simulink model "sgm_iox_io397_pwm_motor_control"  (R2018a)
settings: Solver=FixedStepDiscrete  StartTime=0.0  StopTime=inf  FixedStep=0.001  RelTol=1e-3  EnableMultiTasking=on
undefined symbols (not defined in the file): IO397
libraries: simulink x2, speedgoatlib_fpga_analog_io x1, speedgoatlib_fpga_pwm x1, speedgoatlib_fpga x1
settings Model: SimulationMode=external  ExtModeArmWhenConnect=off  Creator=deastman  LastModifiedBy=daniel.fonte
settings SolverCC: ConcurrentTasks=on  PositivePriorityOrder=on  AutoInsertRateTranBlk=on
settings DataIOCC: LimitDataPoints=on  SaveFormat=StructureWithTime
settings OptimizationCC: BlockReduction=off  OptimizeBlockIOStorage=off  BufferReuse=off  GlobalBufferReuse=off  ExpressionFolding=off  ExpressionDepthLimit=2147483647  LocalBlockOutputs=off  OptimizeDataStoreBuffers=off  BusAssignmentInplaceUpdate=off
settings DebuggingCC: UnderspecifiedInitializationDetection=Classic  MergeDetectMultiDrivingBlocksExec=none  SolverPrmCheckMsg=warning  FcnCallInpInsideContextMsg=warning  AllowSymbolicDim=off  StateNameClashWarn=warning  SFUnexpectedBacktrackingDiag=warning  SFNoUnconditionalDefaultTransitionDiag=warning  SFExecutionAtInitializationDiag=none
settings HardwareCC: ProdBitPerPointer=32  ProdBitPerSizeT=32  ProdBitPerPtrDiffT=32  ProdLargestAtomicFloat=None  ProdWordSize=32  ProdLongLongMode=on  ProdHWDeviceType=Generic->32-bit x86 compatible
settings ModelReferenceCC: PropagateSignalLabelsOutOfModel=off
settings RTWCC: SystemTargetFile=slrt.tlc  TemplateMakefile=slrt_default_tmf  Description=Simulink Real-Time  RTWVerbose=off  Toolchain=Simulink Real-Time Toolchain  BuildConfiguration=Faster Runs  CodeExecutionProfiling=on  RTWCompilerOptimization=on
settings CodeAppCC: StateflowObjectComments=on
settings SimulinkRealTimeCC: SupportVariableSizeSignals=on  RL32LogTETModifier=off  xPCConcurrentTasks=on
settings ConfigComp: CovMetricSettings=dw  CovSaveCumulativeToWorkspaceVar=on  CovSaveSingleToWorkspaceVar=on  CovExternalEMLEnable=off  CovSFcnEnable=off

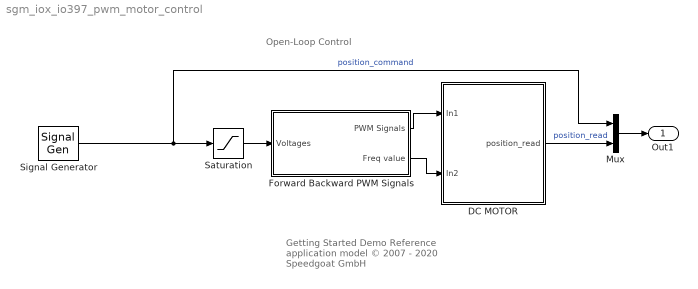
== system sgm_iox_io397_pwm_motor_control ==
  note: Open-Loop Control
  note: Getting Started Demo
      | Reference application model
      | © 2007 - 2020 Speedgoat GmbH
  DC MOTOR : Subsystem
      mask Display: image(imread('hs422.jpg'))
  Forward Backward PWM Signals : Subsystem
      mask init:
      | wave = sin(0:0.4:12);
      | a = length(wave);
      | x1 = linspace(0,8,a);
      | nan1 = NaN(1,2);
      | x2 = x1(end)+[0 1];
      | arrowY = [0 0 0.16 NaN -0.16 0];
      | x3 = x2(end)+[0 2 1.6 NaN 1.6 2];
      | nan2 = NaN(1,2);
      | x4 = x3(end)+[0 1];
      | squareY = [0.5 0 0 0.5 0.5 0 0 0.5 0.5 0 0 0.5 0.5 0 0 0.5 0.5 0 0 0.5 0.5 0];
      | x5 = x4(end)+[0 0 0.4 0.4 0.9 0.9 2.3 2.3 2.6 2.6 3.1 3.1 4.7 4.7 5.4 5.4 5.8 5.8 7.3 7.3 8 8];
      mask Display: plot([x1 x2 x3 x4 x5],[wave nan1 arrowY nan2 squareY])
  Mux : Mux  Inputs=2
  Saturation : Saturate  UpperLimit=5  LowerLimit=-5
  Signal Generator : SignalGenerator  WaveForm=square  Frequency=0.5
  Out1 : Outport
  wires:
  Saturation/1 -> Forward Backward PWM Signals/1(Voltages)
  Forward Backward PWM Signals/1(PWM Signals) -> DC MOTOR/1(In1)
  Mux/1 -> Out1/1
  DC MOTOR/1(position_read) -> Mux/2  "position_read"
  Signal Generator/1 -> Mux/1, Saturation/1  "position_command"
  Forward Backward PWM Signals/2(Freq value) -> DC MOTOR/2(In2)

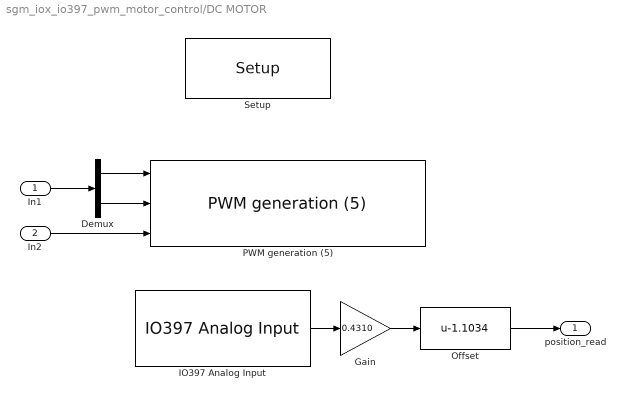
== system sgm_iox_io397_pwm_motor_control/DC MOTOR ==
  In1 : Inport
  In2 : Inport  Port=2
  Demux : Demux  Outputs=2
  Gain : Gain  Gain=0.4310
  IO397 Analog Input : speedgoatlib_fpga_analog_io/IO397 Analog Input  id=1  chan=[1]  range=+5.12 V  trigger=Initiator  ts=0.001  pciSlot=-1  board=IO397-50k
      settings: SourceProductName=Simulink Real-Time: Speedgoat I/O Driver Library
  Offset : Bias  Bias=-1.1034
  PWM generation (5) : speedgoatlib_fpga_pwm/PWM generation (5)  id=1  chan=1  board=IO397-50k  ts=0.001  pciSlot=-1  delay=0  symmetric=Symmetric - PWM generation is centered around half the period  b_is_complement_of_a=Independent of PWM A output  deadband=[0.0]  period=.05  frequency=20  ticks=3749999  a_on=[0]  a_off=[0]  pwm_a_dc=[0.0]  b_on=[0]  b_off=[0]  pwm_b_dc=[0]  c_on=[0.0]  c_off=[0.0]  protection=A/B are forced off when A/B are on.  enable_latch_half_period=off  pwm_update=At period starts  trigger_duration=[100e-6]  trigger_period_start=on  trigger_half_of_the_period=off  trigger_a_on=off  trigger_a_off=off  trigger_b_on=off  trigger_b_off=off  show_a_input=on  show_b_input=on  show_c_input=off  show_period_input=on  show_force_stop_input=off  idle_a=Low when PWM generation is halted  idle_b=Low when PWM generation is halted  idle_c=Low when PWM generation is halted  cancels_pwm_generation=on  invert_a=off  invert_b=off  invert_c=off
      settings: SourceProductName=Simulink Real-Time: Speedgoat I/O Driver Library
  Setup : speedgoatlib_fpga/Setup/Setup  board=IO397-50k  id=1  device_id=1  frontIO=None  rearIO=None  bitstreamFile=speedgoat_IO397_50k_CI_IO397_DUT_DEMO  rev=1.0  timestamp_string=05/10/17 09:15:16  fpgaFreq=75 MHz  fpgaTick=13.33 ns  ProgSpiFlash=off  ProgBPIFlash=off  pciSlot=-1  PullRPort0=pull-up 3.3V  VioPort0=3.3V  PullRPort1=pull-up 3.3V  VioPort1=3.3V  PullRPort2=pull-up 3.3V  VioPort2=3.3V  PullRPort3=pull-up 3.3V  VioPort3=3.3V  PullRPort4=pull-up 3.3V  VioPort4=3.3V  PullRPort5=pull-up 3.3V  VioPort5=3.3V  PullRPort6=pull-up 3.3V  VioPort6=3.3V  PullRPort15=pull-up 3.3V  PullRPort31=pull-up 3.3V  PullRPort47=pull-up 3.3V  PullRPort63=pull-up 3.3V
      settings: SourceProductName=Simulink Real-Time: Speedgoat I/O Driver Library
  position_read : Outport
  wires:
  In1/1 -> Demux/1
  Demux/1 -> PWM generation (5)/1
  Demux/2 -> PWM generation (5)/2
  IO397 Analog Input/1 -> Gain/1
  Offset/1 -> position_read/1
  Gain/1 -> Offset/1
  In2/1 -> PWM generation (5)/3

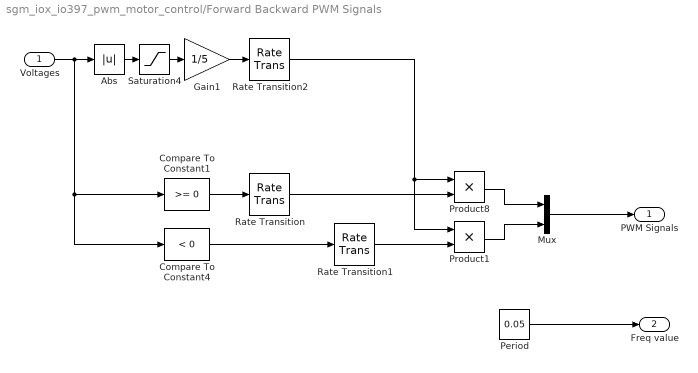
== system sgm_iox_io397_pwm_motor_control/Forward Backward PWM Signals ==
  Voltages : Inport
  Abs : Abs  ZeroCross=off
  Compare To Constant1 : simulink/Logic and Bit Operations/Compare To Constant  relop=>=  const=0  OutDataTypeStr=boolean  ZeroCross=off
  Compare To Constant4 : simulink/Logic and Bit Operations/Compare To Constant  relop=<  const=0  OutDataTypeStr=boolean  ZeroCross=off
  Gain1 : Gain  Gain=1/5
  Mux : Mux  Inputs=2
  Period : Constant  Value=0.05  SampleTime=.01
  Product1 : Product  OutDataTypeStr=double  RndMeth=Zero
  Product8 : Product  OutDataTypeStr=double  RndMeth=Zero
  Rate Transition : RateTransition  Integrity=off  OutPortSampleTimeOpt=Inherit
  Rate Transition1 : RateTransition  Integrity=off  OutPortSampleTimeOpt=Inherit
  Rate Transition2 : RateTransition  Integrity=off  OutPortSampleTimeOpt=Inherit
  Saturation4 : Saturate  UpperLimit=5  LowerLimit=0
  PWM Signals : Outport
  Freq value : Outport  Port=2
  wires:
  Gain1/1 -> Rate Transition2/1
  Abs/1 -> Saturation4/1
  Saturation4/1 -> Gain1/1
  Compare To Constant4/1 -> Rate Transition1/1
  Product1/1 -> Mux/2
  Product8/1 -> Mux/1
  Compare To Constant1/1 -> Rate Transition/1
  Rate Transition2/1 -> Product8/1, Product1/1
  Voltages/1 -> Compare To Constant1/1, Compare To Constant4/1, Abs/1
  Mux/1 -> PWM Signals/1
  Rate Transition/1 -> Product8/2
  Rate Transition1/1 -> Product1/2
  Period/1 -> Freq value/1
